simulink model "lab7_MF_pert"  (R2020a)
settings: Solver=FixedStepAuto  StartTime=0.0  StopTime=400  FixedStep=0.01  RelTol=1e-3
values from neighbouring files (symbols this model uses):
  D = det(A)    [pplane9.m]
undefined symbols (not defined in the file or in its folder): g, h_bar, sigbuilder_block, u_bar
settings Model: Creator=bruno  LastModifiedBy=bruno

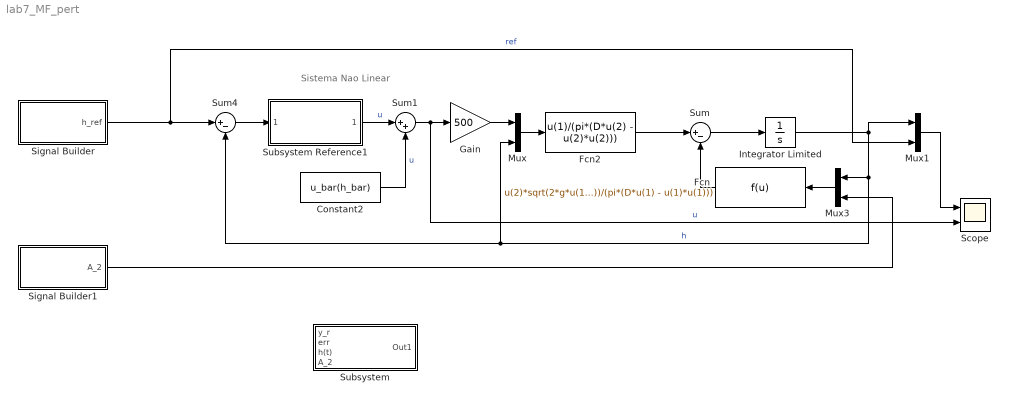
== system lab7_MF_pert ==
  note: Sistema Nao Linear
  Constant2 : Constant  Value=u_bar(h_bar)
  Fcn : Fcn  Expr=u(2)*sqrt(2*g*u(1))/(pi*(D*u(1) - u(1)*u(1)))
  Fcn2 : Fcn  Expr=u(1)/(pi*(D*u(2) - u(2)*u(2)))
  Gain : Gain  Gain=500
  Integrator Limited : Integrator  InitialCondition=h_bar  LimitOutput=on  UpperSaturationLimit=100-0.001  LowerSaturationLimit=0.001
  Mux : Mux  Inputs=2
  Mux1 : Mux  Inputs=2
  Mux3 : Mux  Inputs=2
  Scope : Scope  NumInputPorts=2
  Signal Builder : Subsystem  Tag=STV Subsys  LoadFcn=sigbuilder_block('load');  StartFcn=sigbuilder_block('start');  StopFcn=sigbuilder_block('stop');  ClipboardFcn=sigbuilder_block('clipboard');  mask(Sigbuilder block){tuvar=[0:10]}
      mask help: Simulink:masks:SigbuilderBlock_MD
      mask init:
      | if ~strcmp(get_param(bdroot(gcbh),'SimulationStatus'),'stopped') tuvar = sigbuilder_block('maskInit'); end
      settings: CopyFcn=sigbuilder_block('copy');  DeleteFcn=sigbuilder_block('delete');  ModelCloseFcn=sigbuilder_block('modelClose');  PreSaveFcn=sigbuilder_block('preSave');  PauseFcn=sigbuilder_block('pause');  ContinueFcn=sigbuilder_block('continue');  NameChangeFcn=sigbuilder_block('namechange');  OpenFcn=sigbuilder_block('open',[468 224.25 640.5 336.75 ]);  CloseFcn=sigbuilder_block('close');
      mask Display: plot(0, 0, 100, 100,[2, 2, 32, 32, 2], [68, 8, 8, 68, 68],[32, 2], [38, 38], [32, 19, 2],[53, 60, 44], [32, 17, 17, 2],[16, 16, 31, 31]);txt = getActiveGroup(gcbh);text(2, 100, txt,'verticalAlignment', 'top');
  Signal Builder1 : Subsystem  Tag=STV Subsys  LoadFcn=sigbuilder_block('load');  StartFcn=sigbuilder_block('start');  StopFcn=sigbuilder_block('stop');  ClipboardFcn=sigbuilder_block('clipboard');  mask(Sigbuilder block){tuvar=[0:10]}
      mask help: Simulink:masks:SigbuilderBlock_MD
      mask init:
      | if ~strcmp(get_param(bdroot(gcbh),'SimulationStatus'),'stopped') tuvar = sigbuilder_block('maskInit'); end
      settings: CopyFcn=sigbuilder_block('copy');  DeleteFcn=sigbuilder_block('delete');  ModelCloseFcn=sigbuilder_block('modelClose');  PreSaveFcn=sigbuilder_block('preSave');  PauseFcn=sigbuilder_block('pause');  ContinueFcn=sigbuilder_block('continue');  NameChangeFcn=sigbuilder_block('namechange');  OpenFcn=sigbuilder_block('open',[712.5 235.5 633 342 ]);  CloseFcn=sigbuilder_block('close');
      mask Display: plot(0, 0, 100, 100,[2, 2, 32, 32, 2], [68, 8, 8, 68, 68],[32, 2], [38, 38], [32, 19, 2],[53, 60, 44], [32, 17, 17, 2],[16, 16, 31, 31]);txt = getActiveGroup(gcbh);text(2, 100, txt,'verticalAlignment', 'top');
  Subsystem : Subsystem
  Subsystem Reference1 : Subsystem  ReferencedSubsystem=PID_AW
  Sum : Sum  Inputs=|+-
  Sum1 : Sum  Inputs=|++
  Sum4 : Sum  Inputs=|+-
  wires:
  Sum/1 -> Integrator Limited/1
  Fcn2/1 -> Sum/1
  Fcn/1 -> Sum/2
  Sum1/1 -> Scope/2, Gain/1  "u"
  Integrator Limited/1 -> Mux1/1, Mux/2, Sum4/2, Mux3/1  "h"
  Signal Builder/1(h_ref) -> Mux1/2, Sum4/1  "ref"
  Gain/1 -> Mux/1
  Mux/1 -> Fcn2/1
  Mux1/1 -> Scope/1
  Constant2/1 -> Sum1/2  "u"
  Subsystem Reference1/1 -> Sum1/1  "u"
  Sum4/1 -> Subsystem Reference1/1
  Mux3/1 -> Fcn/1
  Signal Builder1/1(A_2) -> Mux3/2

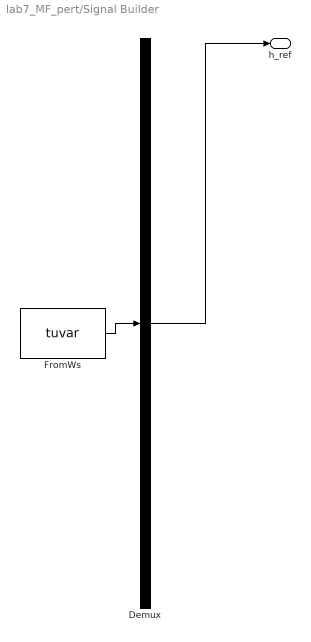
== system lab7_MF_pert/Signal Builder ==
  Demux : Demux  Tag=STV Demux  Outputs=1
      settings: DisplayOption=none
  FromWs : FromWorkspace  Tag=STV FromWs  VariableName=tuvar
      SigBuilderData=|
      | common.afterFinalStr = 'Extrapolate'
      | common.sampleTime = 0
      | dataSet.timeRange = [0 400]
      | dataSet.name = 'Group 1'
      | sbobj.Groups.Name = 'Group 1'
      | sbobj.Groups.Signals.Name = 'h_ref'
      | sbobj.Groups.Signals.XData = [0 50 50 150 150 250 250 300 300 400]
      | sbobj.Groups.Signals.YData = [90 90 50 50 10 10 50 50 90 90]
      | sbobj.Groups.TimeRange = [0 400]
  h_ref : Outport  Tag=STV Outport
  wires:
  Demux/1 -> h_ref/1
  FromWs/1 -> Demux/1

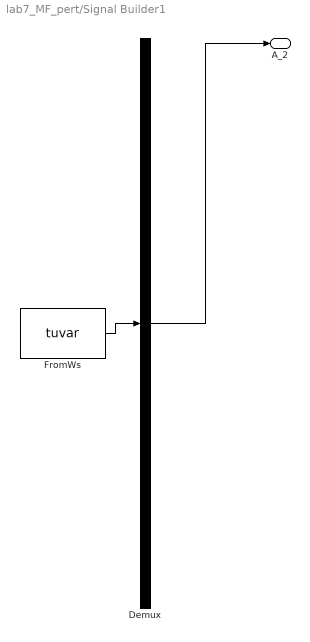
== system lab7_MF_pert/Signal Builder1 ==
  Demux : Demux  Tag=STV Demux  Outputs=1
      settings: DisplayOption=none
  FromWs : FromWorkspace  Tag=STV FromWs  VariableName=tuvar
      SigBuilderData=|
      | common.afterFinalStr = 'Extrapolate'
      | common.sampleTime = 0
      | dataSet.timeRange = [0 400]
      | dataSet.name = 'Group 1'
      | sbobj.Groups.Name = 'Group 1'
      | sbobj.Groups.Signals.Name = 'A_2'
      | sbobj.Groups.Signals.XData = [0 50 150 250 300 350 350 375 375 400]
      | sbobj.Groups.Signals.YData = [19.6 19.6 19.6 19.6 19.6 19.6 0 0 15 15]
      | sbobj.Groups.TimeRange = [0 400]
  A_2 : Outport  Tag=STV Outport
  wires:
  Demux/1 -> A_2/1
  FromWs/1 -> Demux/1

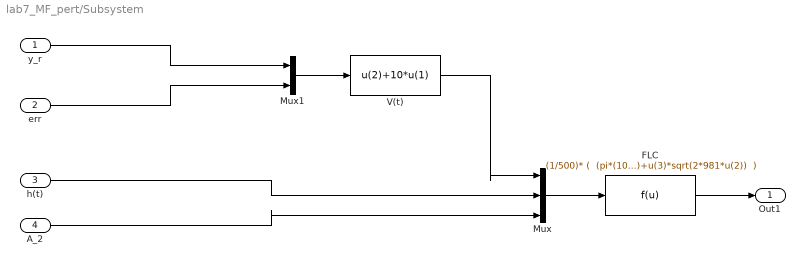
== system lab7_MF_pert/Subsystem ==
  y_r : Inport
  err : Inport  Port=2
  h(t) : Inport  Port=3
  A_2 : Inport  Port=4
  FLC : Fcn  Expr="(1/500)* (  (pi*(100*u(2)-u(2)^2)) *u(1)+u(3)*sqrt(2*981*u(2))  )"
  Mux : Mux  Inputs=3
  Mux1 : Mux  Inputs=2
  V(t) : Fcn  Expr=u(2)+10*u(1)
  Out1 : Outport
  wires:
  FLC/1 -> Out1/1
  Mux/1 -> FLC/1
  V(t)/1 -> Mux/1
  A_2/1 -> Mux/3
  h(t)/1 -> Mux/2
  Mux1/1 -> V(t)/1
  y_r/1 -> Mux1/1
  err/1 -> Mux1/2
